simulink model "kalman_vector_oscillator_2021_04_22"  (R2020a)
settings: Solver=ode23tb  StartTime=0.0  StopTime=simlength  MaxStep=Ts
values from neighbouring files (symbols this model uses):
  Afd = [exp(-Ts*w)*(1+Ts*w) exp(-Ts*w)*Ts; -exp(-Ts*w)*Ts*w^2 exp(-Ts*w)*(1-Ts*w)]    [init_oscillator_2021_03_26.m]
  Bfd = [(1-exp(-Ts*w)*(1+Ts*w))/w^2 exp(-Ts*w)*Ts]'    [init_oscillator_2021_03_26.m]
  Cf = [2*w^2 0]    [init_oscillator_2021_03_26.m]
  ki = 2    [init_oscillator_2021_03_26.m]
  kp = 1    [init_oscillator_2021_03_26.m]
  q1kalman = Ts/10    (= 1e-05)    [init_oscillator_2021_03_26.m]
  q2kalman = Ts/10    (= 1e-05)    [init_oscillator_2021_03_26.m]
  Rkalman = 0.1/q1kalman    (= 10000)    [init_oscillator_2021_03_26.m]
  Tc = 1e-5    (= 1e-05)    [init_oscillator_2021_03_26.m]
  Ts = 1/10e3    (= 0.0001)    [init_oscillator_2021_03_26.m]
  w = 2*pi*f    (= 314.159265359)    [init_oscillator_2021_03_26.m]
libraries: simulink x1, cstblocks x1
settings Model: SimulationMode=accelerator  Creator=dbagn  LastModifiedBy=dbagn
settings SolverCC: SolverResetMethod=Robust
settings DataIOCC: ReturnWorkspaceOutputs=off

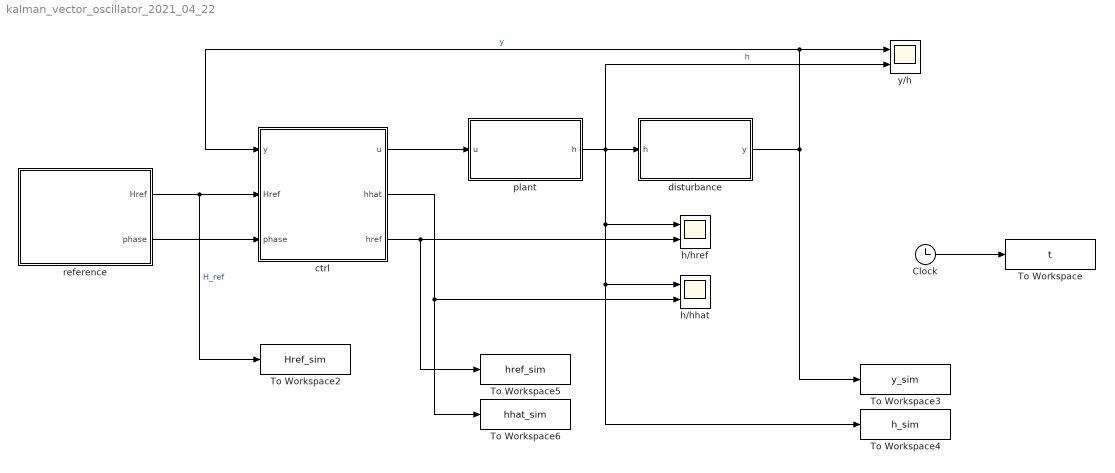
== system kalman_vector_oscillator_2021_04_22 ==
  Clock : Clock
  To Workspace : ToWorkspace  VariableName=t  SampleTime=Tc
      settings: MaxDataPoints=Nc
  To Workspace2 : ToWorkspace  VariableName=Href_sim  SampleTime=Tc
      settings: MaxDataPoints=Nc
  To Workspace3 : ToWorkspace  VariableName=y_sim  SampleTime=Tc
      settings: MaxDataPoints=Nc
  To Workspace4 : ToWorkspace  VariableName=h_sim  SampleTime=Tc
      settings: MaxDataPoints=Nc
  To Workspace5 : ToWorkspace  VariableName=href_sim  SampleTime=Tc
      settings: MaxDataPoints=Nc
  To Workspace6 : ToWorkspace  VariableName=hhat_sim  SampleTime=Tc
      settings: MaxDataPoints=Nc
  ctrl : Subsystem
  disturbance : Subsystem
  h/hhat : Scope  NumInputPorts=2
  h/href : Scope  NumInputPorts=2
  plant : Subsystem
  reference : Subsystem
  y/h : Scope  NumInputPorts=2
  wires:
  reference/1(Href) -> To Workspace2/1, ctrl/2(Href)  "H_ref"
  ctrl/1(u) -> plant/1(u)
  reference/2(phase) -> ctrl/3(phase)
  ctrl/3(href) -> h/href/2, To Workspace5/1
  ctrl/2(hhat) -> To Workspace6/1, h/hhat/2
  Clock/1 -> To Workspace/1
  plant/1(h) -> To Workspace4/1, h/hhat/1, h/href/1, y/h/2, disturbance/1(h)  "h"
  disturbance/1(y) -> To Workspace3/1, ctrl/1(y), y/h/1  "y"

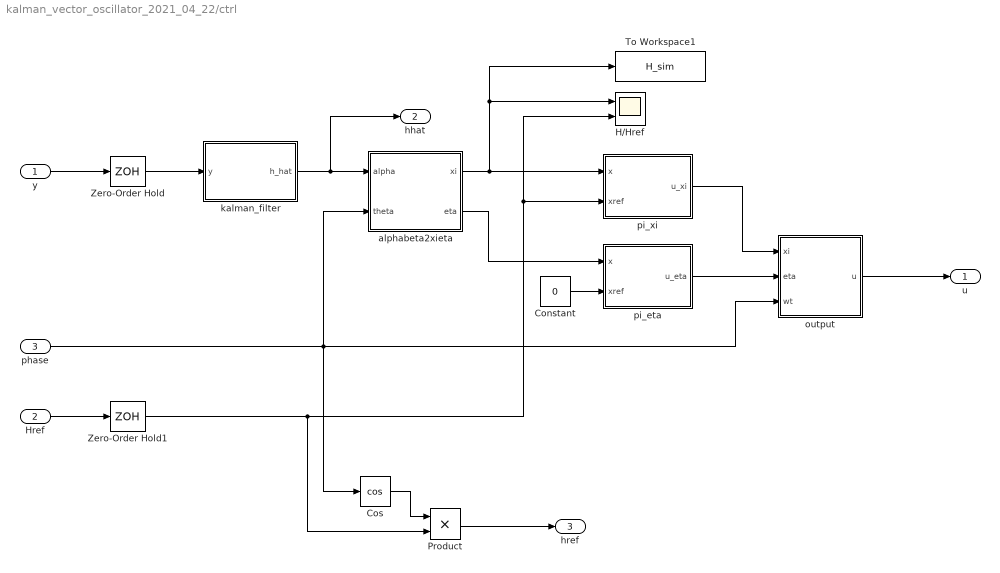
== system kalman_vector_oscillator_2021_04_22/ctrl ==
  y : Inport
  Href : Inport  Port=2
  phase : Inport  Port=3
  Constant : Constant  Value=0
  Cos : Trigonometry  Operator=cos
  H/Href : Scope  NumInputPorts=2
  Product : Product
  To Workspace1 : ToWorkspace  VariableName=H_sim  SampleTime=Tc
      settings: MaxDataPoints=Nc
  Zero-Order Hold : ZeroOrderHold  SampleTime=Ts
  Zero-Order Hold1 : ZeroOrderHold  SampleTime=Ts
  alphabeta2xieta : Subsystem
  kalman_filter : Subsystem
  output : Subsystem
  "pi_eta " : Subsystem  mask{kp=kp, ki=ki, ts=Ts, sat_pos=inf, sat_neg=-inf}
  pi_xi : Subsystem  mask{kp=kp, ki=ki, ts=Ts, sat_pos=inf, sat_neg=-inf}
  u : Outport  VectorParamsAs1DForOutWhenUnconnected=off
  hhat : Outport  Port=2  VectorParamsAs1DForOutWhenUnconnected=off
  href : Outport  Port=3  VectorParamsAs1DForOutWhenUnconnected=off
  wires:
  Href/1 -> Zero-Order Hold1/1
  y/1 -> Zero-Order Hold/1
  output/1(u) -> u/1
  Zero-Order Hold/1 -> kalman_filter/1(y)
  phase/1 -> alphabeta2xieta/2(theta), output/3(wt), Cos/1
  alphabeta2xieta/1(xi) -> To Workspace1/1, H/Href/1, pi_xi/1(x)
  Zero-Order Hold1/1 -> Product/2, H/Href/2, pi_xi/2(xref)
  alphabeta2xieta/2(eta) -> "pi_eta "/1(x)
  Cos/1 -> Product/1
  Product/1 -> href/1
  Constant/1 -> "pi_eta "/2(xref)
  kalman_filter/1(h_hat) -> hhat/1, alphabeta2xieta/1(alpha)
  pi_xi/1(u_xi) -> output/1(xi)
  "pi_eta "/1(u_eta) -> output/2(eta)

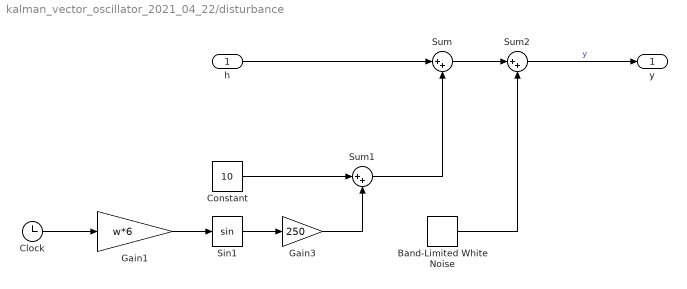
== system kalman_vector_oscillator_2021_04_22/disturbance ==
  h : Inport
  Band-Limited White Noise : simulink/Sources/Band-Limited White Noise  Cov=10*Tc  Ts=Tc  seed=[23341]
  Clock : Clock
  Constant : Constant  Value=10
  Gain1 : Gain  Gain=w*6
  Gain3 : Gain  Gain=250
  Sin1 : Trigonometry
  Sum : Sum  Inputs=|++
  Sum1 : Sum  Inputs=|++
  Sum2 : Sum  Inputs=|++
  y : Outport
  wires:
  Gain3/1 -> Sum1/2
  Band-Limited White Noise/1 -> Sum2/2
  Sin1/1 -> Gain3/1
  Clock/1 -> Gain1/1
  Sum/1 -> Sum2/1
  Constant/1 -> Sum1/1
  Sum2/1 -> y/1  "y"
  Gain1/1 -> Sin1/1
  h/1 -> Sum/1
  Sum1/1 -> Sum/2

== system kalman_vector_oscillator_2021_04_22/plant ==
  u : Inport
  LTI System : cstblocks/LTI System  sys=plant  IC=[]
  h : Outport  VectorParamsAs1DForOutWhenUnconnected=off
  wires:
  LTI System/1 -> h/1
  u/1 -> LTI System/1

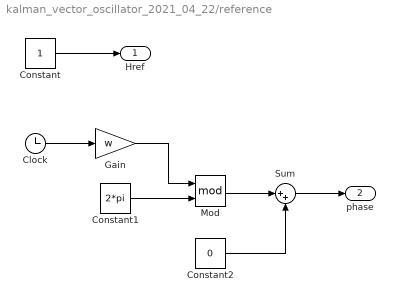
== system kalman_vector_oscillator_2021_04_22/reference ==
  Clock : Clock
  Constant : Constant
  Constant1 : Constant  Value=2*pi
  Constant2 : Constant  Value=0
  Gain : Gain  Gain=w
  Mod : Math  Operator=mod  SaturateOnIntegerOverflow=on
  Sum : Sum  Inputs=|++
  Href : Outport
  phase : Outport  Port=2
  wires:
  Clock/1 -> Gain/1
  Constant/1 -> Href/1
  Constant1/1 -> Mod/2
  Gain/1 -> Mod/1
  Mod/1 -> Sum/1
  Sum/1 -> phase/1
  Constant2/1 -> Sum/2

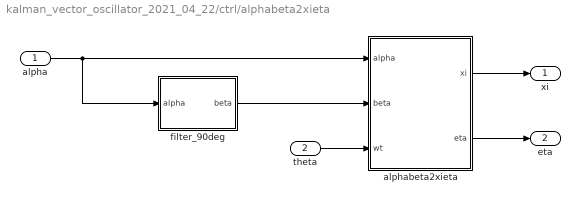
== system kalman_vector_oscillator_2021_04_22/ctrl/alphabeta2xieta ==
  alpha : Inport
  theta : Inport  Port=2
  alphabeta2xieta : Subsystem
  filter_90deg : Subsystem
  xi : Outport
  eta : Outport  Port=2
  wires:
  alpha/1 -> alphabeta2xieta/1(alpha), filter_90deg/1(alpha)
  filter_90deg/1(beta) -> alphabeta2xieta/2(beta)
  theta/1 -> alphabeta2xieta/3(wt)
  alphabeta2xieta/1(xi) -> xi/1
  alphabeta2xieta/2(eta) -> eta/1

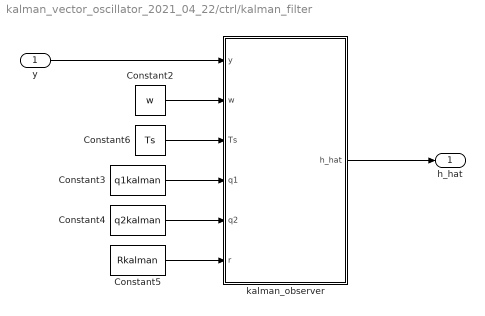
== system kalman_vector_oscillator_2021_04_22/ctrl/kalman_filter ==
  y : Inport
  Constant2 : Constant  Value=w
  Constant3 : Constant  Value=q1kalman
  Constant4 : Constant  Value=q2kalman
  Constant5 : Constant  Value=Rkalman
  Constant6 : Constant  Value=Ts
  kalman_observer : MATLAB Function  TreatAsAtomicUnit=on  SystemSampleTime=Ts
  h_hat : Outport
  wires:
  Constant2/1 -> kalman_observer/2(w)
  y/1 -> kalman_observer/1(y)
  Constant6/1 -> kalman_observer/3(Ts)
  Constant5/1 -> kalman_observer/6(r)
  Constant3/1 -> kalman_observer/4(q1)
  Constant4/1 -> kalman_observer/5(q2)
  kalman_observer/1(h_hat) -> h_hat/1

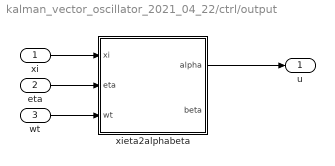
== system kalman_vector_oscillator_2021_04_22/ctrl/output ==
  xi : Inport
  eta : Inport  Port=2
  wt : Inport  Port=3
  xieta2alphabeta : Subsystem
  u : Outport  VectorParamsAs1DForOutWhenUnconnected=off
  wires:
  xi/1 -> xieta2alphabeta/1(xi)
  eta/1 -> xieta2alphabeta/2(eta)
  wt/1 -> xieta2alphabeta/3(wt)
  xieta2alphabeta/1(alpha) -> u/1

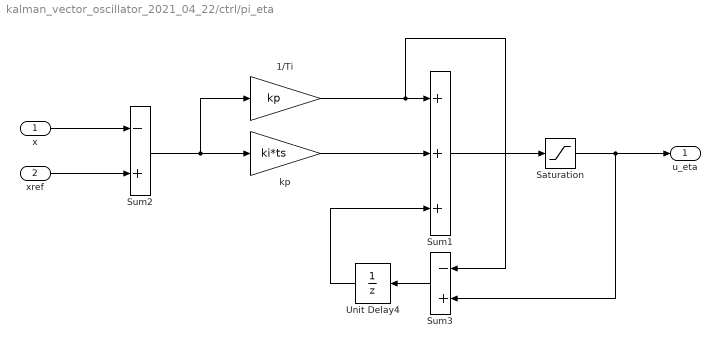
== system kalman_vector_oscillator_2021_04_22/ctrl/pi_eta  ==
  x : Inport
  xref : Inport  Port=2
  1/Ti : Gain  Gain=kp  SaturateOnIntegerOverflow=on  OutDataTypeStr=Inherit: Same as input  ParamDataTypeStr=Inherit: Same as input
  Saturation : Saturate  UpperLimit=sat_pos  LowerLimit=sat_neg
  Sum1 : Sum  Inputs=+++  SaturateOnIntegerOverflow=on
  Sum2 : Sum  Inputs=-+  SaturateOnIntegerOverflow=on
  Sum3 : Sum  Inputs=-+  SaturateOnIntegerOverflow=on
  Unit Delay4 : UnitDelay  SampleTime=ts  HasFrameUpgradeWarning=on
  kp : Gain  Gain=ki*ts  SaturateOnIntegerOverflow=on  OutDataTypeStr=Inherit: Same as input  ParamDataTypeStr=Inherit: Same as input
  u_eta : Outport
  wires:
  Saturation/1 -> Sum3/2, u_eta/1
  Unit Delay4/1 -> Sum1/3
  Sum1/1 -> Saturation/1
  x/1 -> Sum2/1
  Sum3/1 -> Unit Delay4/1
  1/Ti/1 -> Sum3/1, Sum1/1
  Sum2/1 -> 1/Ti/1, kp/1
  kp/1 -> Sum1/2
  xref/1 -> Sum2/2

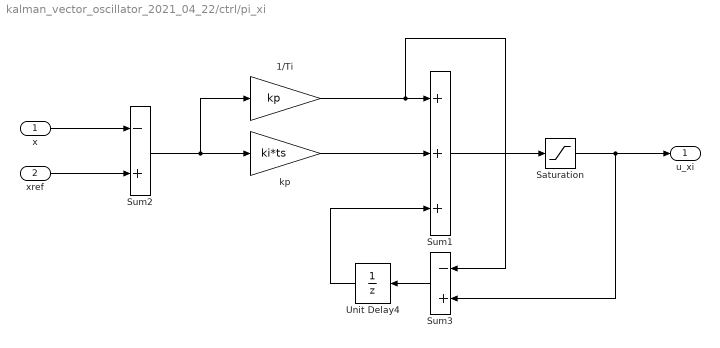
== system kalman_vector_oscillator_2021_04_22/ctrl/pi_xi ==
  x : Inport
  xref : Inport  Port=2
  1/Ti : Gain  Gain=kp  SaturateOnIntegerOverflow=on  OutDataTypeStr=Inherit: Same as input  ParamDataTypeStr=Inherit: Same as input
  Saturation : Saturate  UpperLimit=sat_pos  LowerLimit=sat_neg
  Sum1 : Sum  Inputs=+++  SaturateOnIntegerOverflow=on
  Sum2 : Sum  Inputs=-+  SaturateOnIntegerOverflow=on
  Sum3 : Sum  Inputs=-+  SaturateOnIntegerOverflow=on
  Unit Delay4 : UnitDelay  SampleTime=ts  HasFrameUpgradeWarning=on
  kp : Gain  Gain=ki*ts  SaturateOnIntegerOverflow=on  OutDataTypeStr=Inherit: Same as input  ParamDataTypeStr=Inherit: Same as input
  u_xi : Outport
  wires:
  xref/1 -> Sum2/2
  kp/1 -> Sum1/2
  Sum2/1 -> kp/1, 1/Ti/1
  1/Ti/1 -> Sum1/1, Sum3/1
  Sum3/1 -> Unit Delay4/1
  x/1 -> Sum2/1
  Sum1/1 -> Saturation/1
  Unit Delay4/1 -> Sum1/3
  Saturation/1 -> u_xi/1, Sum3/2

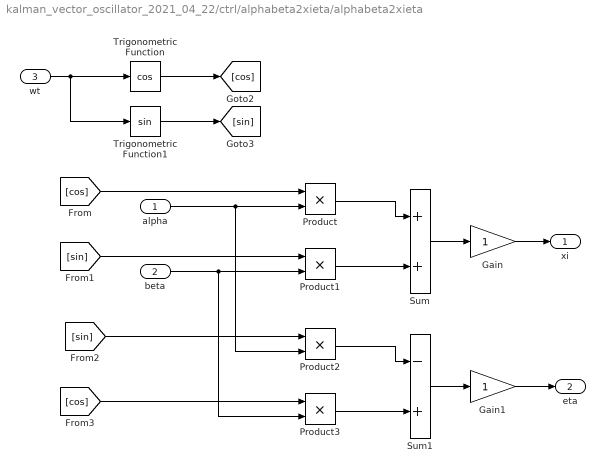
== system kalman_vector_oscillator_2021_04_22/ctrl/alphabeta2xieta/alphabeta2xieta ==
  alpha : Inport
  beta : Inport  Port=2
  wt : Inport  Port=3
  Gain : Gain
  Gain1 : Gain
  Product{,1..3} (4 alike) : Product  RndMeth=Zero
  Sum : Sum
  Sum1 : Sum  Inputs=-+
  Trigonometric Function : Trigonometry  Operator=cos
  Trigonometric Function1 : Trigonometry
  xi : Outport  VectorParamsAs1DForOutWhenUnconnected=off
  eta : Outport  Port=2  VectorParamsAs1DForOutWhenUnconnected=off
  wires:
  wt/1 -> Trigonometric Function1/1, Trigonometric Function/1
  Trigonometric Function/1 -> [cos]
  Trigonometric Function1/1 -> [sin]
  Gain1/1 -> eta/1
  Gain/1 -> xi/1
  Sum1/1 -> Gain1/1
  [cos] -> Product3/1
  Product3/1 -> Sum1/2
  Product2/1 -> Sum1/1
  [sin] -> Product2/1
  Sum/1 -> Gain/1
  beta/1 -> Product1/2, Product3/2
  [sin] -> Product1/1
  Product1/1 -> Sum/2
  Product/1 -> Sum/1
  alpha/1 -> Product2/2, Product/2
  [cos] -> Product/1

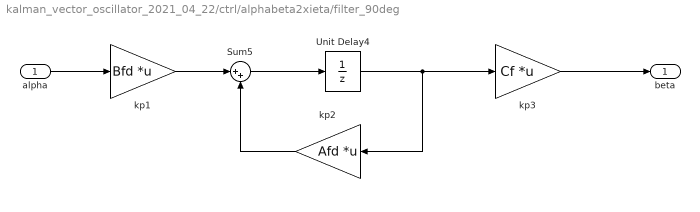
== system kalman_vector_oscillator_2021_04_22/ctrl/alphabeta2xieta/filter_90deg ==
  alpha : Inport
  Sum5 : Sum  Inputs=|++
  Unit Delay4 : UnitDelay  SampleTime=Ts  HasFrameUpgradeWarning=on
  kp1 : Gain  Gain=Bfd  Multiplication=Matrix(K*u)  SaturateOnIntegerOverflow=on  OutDataTypeStr=Inherit: Same as input  ParamDataTypeStr=Inherit: Same as input
  kp2 : Gain  Gain=Afd  Multiplication=Matrix(K*u)  SaturateOnIntegerOverflow=on  OutDataTypeStr=Inherit: Same as input  ParamDataTypeStr=Inherit: Same as input
  kp3 : Gain  Gain=Cf  Multiplication=Matrix(K*u)  SaturateOnIntegerOverflow=on  OutDataTypeStr=Inherit: Same as input  ParamDataTypeStr=Inherit: Same as input
  beta : Outport
  wires:
  Unit Delay4/1 -> kp2/1, kp3/1
  Sum5/1 -> Unit Delay4/1
  kp3/1 -> beta/1
  kp2/1 -> Sum5/2
  kp1/1 -> Sum5/1
  alpha/1 -> kp1/1

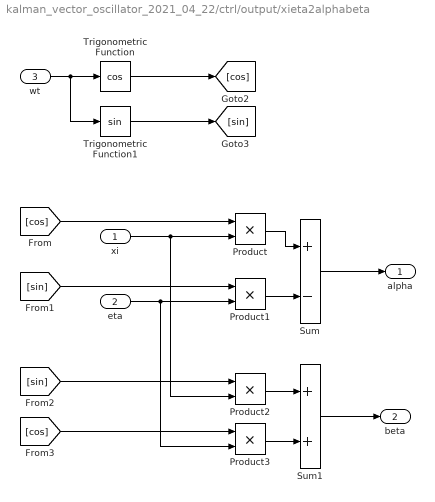
== system kalman_vector_oscillator_2021_04_22/ctrl/output/xieta2alphabeta ==
  xi : Inport
  eta : Inport  Port=2
  wt : Inport  Port=3
  Product{,1..3} (4 alike) : Product  RndMeth=Zero
  Sum : Sum  Inputs=+-
  Sum1 : Sum
  Trigonometric Function : Trigonometry  Operator=cos
  Trigonometric Function1 : Trigonometry
  alpha : Outport  VectorParamsAs1DForOutWhenUnconnected=off
  beta : Outport  Port=2  VectorParamsAs1DForOutWhenUnconnected=off
  wires:
  Sum1/1 -> beta/1
  [cos] -> Product3/1
  Product3/1 -> Sum1/2
  Product2/1 -> Sum1/1
  [sin] -> Product2/1
  Sum/1 -> alpha/1
  eta/1 -> Product3/2, Product1/2
  [sin] -> Product1/1
  Product1/1 -> Sum/2
  Product/1 -> Sum/1
  xi/1 -> Product2/2, Product/2
  [cos] -> Product/1
  Trigonometric Function1/1 -> [sin]
  Trigonometric Function/1 -> [cos]
  wt/1 -> Trigonometric Function/1, Trigonometric Function1/1

== matlab function kalman_vector_oscillator_2021_04_22/ctrl/kalman_filter/kalman_observer ==
  data: y input; h_hat output; w input; Ts input; q1 input; q2 input; r input
function h_hat   = KFO(y,w,Ts,q1,q2,r)

    persistent   x1_po x2_po p11_po p12_po p21_po p22_po

    if isempty(x1_po)
        x1_po = 0;
        x2_po = 0;
        p11_po = 0;
        p12_po = 0;
        p21_po = 0;
        p22_po = 0;        
    end
    
    a11 = cos(w*Ts);
    a12 = sin(w*Ts);
    a21 = -sin(w*Ts);
    a22 = cos(w*Ts);
   
    
    
    x1_pr = a11*x1_po + a12*x2_po;
    x2_pr = a21*x1_po + a22*x2_po;
    
    p11_pr = q1 + a11*(a11*p11_po+a12*p21_po) + a12*(a11*p12_po+a12*p22_po);
    p12_pr = a21*(a11*p11_po+a12*p21_po) + a22*(a11*p12_po+a12*p22_po);
    p21_pr = a11*(a21*p11_po+a22*p21_po) + a12*(a21*p12_po+a22*p22_po);
    p22_pr = q2 + a21*(a21*p11_po+a22*p21_po) + a22*(a21*p12_po+a22*p22_po);
    
    l1 = p11_pr/(p11_pr + r);
    l2 = p21_pr/(p11_pr + r);
    
    x1_po = x1_pr + l1*(y-x1_pr);
    x2_po = x2_pr + l2*(y-x1_pr);
    
    p11_po = (1-l1)*p11_pr;
    p12_po = (1-l1)*p12_pr;
    p21_po = p21_pr-l2*p11_pr;
    p22_po = p22_pr-l2*p12_pr;
    
    
    
    h_hat = x1_pr;
end
